simulink library "INT_OilT_DD"  (R2016b)
settings: Solver=VariableStepAuto  StartTime=0.0  StopTime=10.0  RelTol=1e-3
settings Model: Creator=Administrator  LastModifiedBy=Administrator

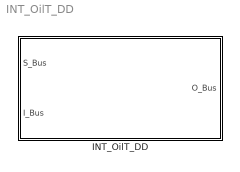
== system INT_OilT_DD ==
  INT_OilT_DD : Subsystem

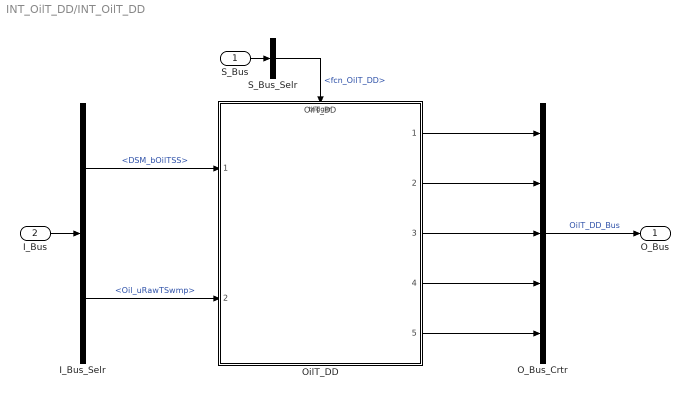
== system INT_OilT_DD/INT_OilT_DD ==
  S_Bus : Inport
  I_Bus : Inport  Port=2
  I_Bus_Selr : BusSelector  OutputSignals=DSM_bOilTSS,Oil_uRawTSwmp
  O_Bus_Crtr : BusCreator  Inputs=5
  OilT_DD : ModelReference  ModelNameDialog=OilT_DD  SimulationMode=Normal  ModelReferenceVersion=1.2  TriggerPortName=function  TriggerPortTriggerType=function-call  TriggerPortStatesWhenEnabling=held
  S_Bus_Selr : BusSelector  OutputSignals=fcn_OilT_DD
  O_Bus : Outport
  wires:
  S_Bus_Selr/1 -> OilT_DD/Trigger  "<fcn_OilT_DD>"
  S_Bus/1 -> S_Bus_Selr/1
  I_Bus/1 -> I_Bus_Selr/1
  I_Bus_Selr/1 -> OilT_DD/1  "<DSM_bOilTSS>"
  I_Bus_Selr/2 -> OilT_DD/2  "<Oil_uRawTSwmp>"
  O_Bus_Crtr/1 -> O_Bus/1  "OilT_DD_Bus"
  OilT_DD/1 -> O_Bus_Crtr/1
  OilT_DD/2 -> O_Bus_Crtr/2
  OilT_DD/3 -> O_Bus_Crtr/3
  OilT_DD/4 -> O_Bus_Crtr/4
  OilT_DD/5 -> O_Bus_Crtr/5
